simulink model "controller"  (Simulink 7.3)
settings: Solver=FixedStepDiscrete  StartTime=0.0  StopTime=inf  FixedStep=900  RelTol=1e-3
libraries: simulink x6
settings Model: Creator=mwetter  LastModifiedBy=mwetter  ExtModeAutoUpdateStatusClock=off
settings OptimizationCC: InitFltsAndDblsToZero=on
settings DebuggingCC: SaveWithParameterizedLinksMsg=none
settings GRTTargetCC: TargetFcnLib=ansi_tfl_tmw.mat

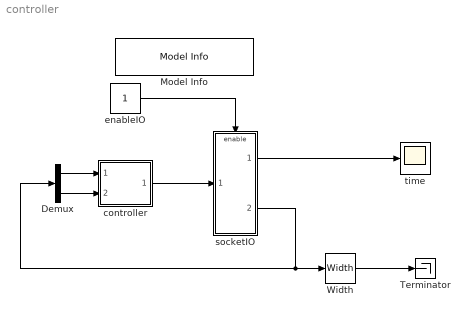
== system controller ==
  Demux : Demux  Outputs=2
  Model Info : simulink/Model-Wide Utilities/Model Info  SystemSampleTime=-1  InitialBlockCM=None  BlockCM=None  Frame=off  DisplayStringWithTags=|  HorizontalTextAlignment=Left  LeftAlignmentValue=0.02  SourceBlockDiagram=controller  TagMaxNumber=20
      | Model Info
      | % Set to 1 to enable IO
  Terminator : Terminator
  Width : Width  DataType=int16
  controller : Subsystem
  enableIO : Constant  OutDataType=sfix(16)  OutScaling=2^0
  socketIO : Subsystem
  time : Scope
  wires:
  socketIO/2(dblOut) -> Width/1, Demux/1
  socketIO/1(simTim) -> time/1
  Width/1 -> Terminator/1
  enableIO/1 -> socketIO/Enable
  Demux/1 -> controller/1(time)
  Demux/2 -> controller/2(TOut)
  controller/1(TSet) -> socketIO/1(dblIn)

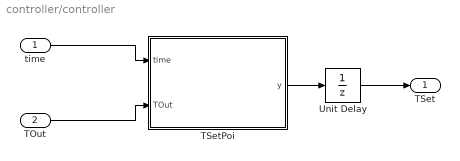
== system controller/controller ==
  time : Inport
  TOut : Inport  Port=2
  TSetPoi : Subsystem
  Unit Delay : UnitDelay  X0=[20, 25]  SampleTime=-1
  TSet : Outport
  wires:
  time/1 -> TSetPoi/1(time)
  TOut/1 -> TSetPoi/2(TOut)
  Unit Delay/1 -> TSet/1
  TSetPoi/1(y) -> Unit Delay/1

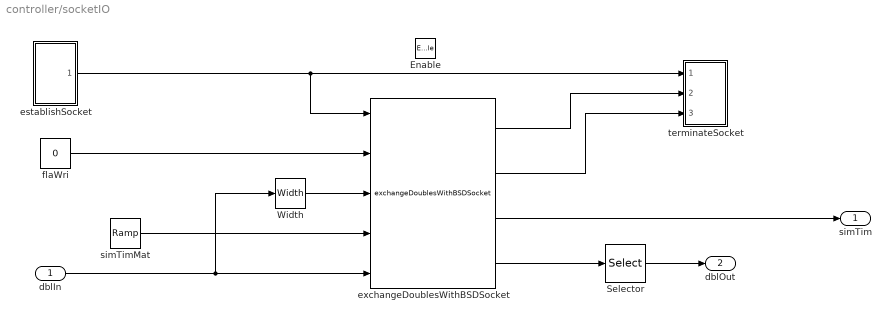
== system controller/socketIO ==
  dblIn : Inport
  Enable : EnablePort
  Selector : Selector  InputPortWidth=128  IndexOptions=Index vector (dialog)  Indices=[1 2]  OutputSizes=1
  Width : Width  DataType=int16
  establishSocket : Subsystem  TreatAsAtomicUnit=on
  exchangeDoublesWithBSDSocket : S-Function  FunctionName=exchangeDoublesWithBSDSocket  EnableBusSupport=off  mask(Legacy Function){SFunctionSpec=int16 y1 = exchangeDoublesWithBSDSocket(int16 u1[1], int16 u2[1], int16 y2[1], double u3[1], double u4[], double y3[1], double y4[50]), ShowSpec=off}
      mask prompts: ShowSpec "Display function specification"
      mask help:
      | This block allows the user to call the following C function(s) in Simulink:
      |
      |  InitializeConditionsFcn: none
      |
      |  StartFcn: none
      |
      |  OutputFcn: int16 y1 = exchangeDoublesWithBSDSocket(int16 u1[1], int16 u2[1], int16 y2[1], double u3[1], double u4[], double y3[1], double y4[50])
      |
      |  TerminateFcn: none
      mask CallbackString:
      | |if strcmp(get_param(gcbh, 'ShowSpec'), 'on')
      |   set_param(gcbh, 'MaskDisplay', sprintf('fprintf(''%s'');', get_param(gcbh, 'SFunctionSpec')));
      | else
      |   set_param(gcbh, 'MaskDisplay', sprintf('fprintf(''%s'');', get_param(gcbh, 'FunctionName')));
      | end
      mask Display: fprintf('exchangeDoublesWithBSDSocket');
  flaWri : Constant  Value=0  OutDataTypeMode=int16  OutDataType=sfix(16)  OutScaling=2^0  OutDataTypeStr=int16
  simTimMat : simulink/Sources/Ramp  SystemSampleTime=-1  slope=1  start=0  X0=0
  terminateSocket : Subsystem
  simTim : Outport
  dblOut : Outport  Port=2
  wires:
  establishSocket/1(socketFD) -> exchangeDoublesWithBSDSocket/1, terminateSocket/1(sockfd)
  flaWri/1 -> exchangeDoublesWithBSDSocket/2
  exchangeDoublesWithBSDSocket/3 -> simTim/1
  dblIn/1 -> exchangeDoublesWithBSDSocket/5, Width/1
  simTimMat/1 -> exchangeDoublesWithBSDSocket/4
  Width/1 -> exchangeDoublesWithBSDSocket/3
  Selector/1 -> dblOut/1
  exchangeDoublesWithBSDSocket/4 -> Selector/1
  exchangeDoublesWithBSDSocket/1 -> terminateSocket/2(excRetVal)
  exchangeDoublesWithBSDSocket/2 -> terminateSocket/3(excFlaRea)

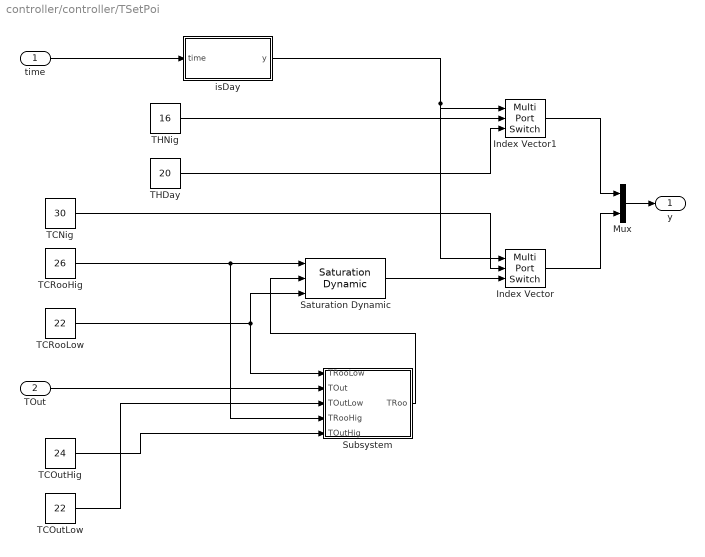
== system controller/controller/TSetPoi ==
  time : Inport  OutDataType=sfix(16)  OutScaling=2^0
  TOut : Inport  Port=2  OutDataType=sfix(16)  OutScaling=2^0
  Index Vector : MultiPortSwitch  Inputs=2  zeroidx=on  OutDataType=sfix(16)  OutScaling=2^0
  Index Vector1 : MultiPortSwitch  Inputs=2  zeroidx=on  OutDataType=sfix(16)  OutScaling=2^0
  Mux : Mux  Inputs=2
  Saturation Dynamic : simulink/Discontinuities/Saturation Dynamic  SystemSampleTime=-1  OutMin=[]  OutMax=[]  OutDataTypeStr=Inherit: Same as second input  OutDataType=sfix(16)  OutScaling=2^-10  DoSatur=off
  Subsystem : Subsystem
  TCNig : Constant  Value=30  OutDataType=sfix(16)  OutScaling=2^0
  TCOutHig : Constant  Value=24  OutDataType=sfix(16)  OutScaling=2^0
  TCOutLow : Constant  Value=22  OutDataType=sfix(16)  OutScaling=2^0
  TCRooHig : Constant  Value=26  OutDataType=sfix(16)  OutScaling=2^0
  TCRooLow : Constant  Value=22  OutDataType=sfix(16)  OutScaling=2^0
  THDay : Constant  Value=20  OutDataType=sfix(16)  OutScaling=2^0
  THNig : Constant  Value=16  OutDataType=sfix(16)  OutScaling=2^0
  isDay : Subsystem
  y : Outport  OutDataType=sfix(16)  OutScaling=2^0
  wires:
  TOut/1 -> Subsystem/2(TOut)
  TCOutLow/1 -> Subsystem/3(TOutLow)
  TCOutHig/1 -> Subsystem/5(TOutHig)
  TCRooHig/1 -> Saturation Dynamic/1, Subsystem/4(TRooHig)
  TCRooLow/1 -> Saturation Dynamic/3, Subsystem/1(TRooLow)
  time/1 -> isDay/1(time)
  isDay/1(y) -> Index Vector/1, Index Vector1/1
  TCNig/1 -> Index Vector/2
  Subsystem/1(TRoo) -> Saturation Dynamic/2
  Saturation Dynamic/1 -> Index Vector/3
  THNig/1 -> Index Vector1/2
  THDay/1 -> Index Vector1/3
  Index Vector1/1 -> Mux/1
  Index Vector/1 -> Mux/2
  Mux/1 -> y/1

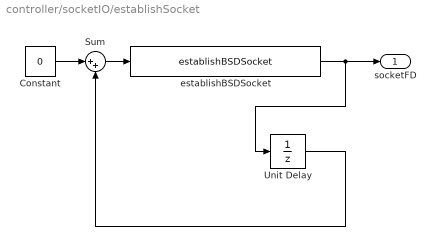
== system controller/socketIO/establishSocket ==
  Constant : Constant  Value=0  OutDataTypeMode=int16  OutDataType=sfix(16)  OutScaling=2^0  OutDataTypeStr=int16
  Sum : Sum  Inputs=|++  OutDataType=sfix(16)  OutScaling=2^0
  Unit Delay : UnitDelay  SampleTime=-1
  establishBSDSocket : S-Function  FunctionName=establishBSDSocket  EnableBusSupport=off  mask(Legacy Function){SFunctionSpec=int16 y1 = establishBSDSocket(void), ShowSpec=on}
      mask prompts: ShowSpec "Display function specification"
      mask help:
      | This block allows the user to call the following C function(s) in Simulink:
      |
      |  InitializeConditionsFcn: none
      |
      |  StartFcn: none
      |
      |  OutputFcn: int16 y1 = establishBSDSocket(void)
      |
      |  TerminateFcn: none
      mask CallbackString:
      | |if strcmp(get_param(gcbh, 'ShowSpec'), 'on')
      |   set_param(gcbh, 'MaskDisplay', sprintf('fprintf(''%s'');', get_param(gcbh, 'SFunctionSpec')));
      | else
      |   set_param(gcbh, 'MaskDisplay', sprintf('fprintf(''%s'');', get_param(gcbh, 'FunctionName')));
      | end
      mask Display: fprintf('int16 y1 = establishBSDSocket(void)');
  socketFD : Outport
  wires:
  establishBSDSocket/1 -> socketFD/1, Unit Delay/1
  Unit Delay/1 -> Sum/2
  Constant/1 -> Sum/1
  Sum/1 -> establishBSDSocket/1

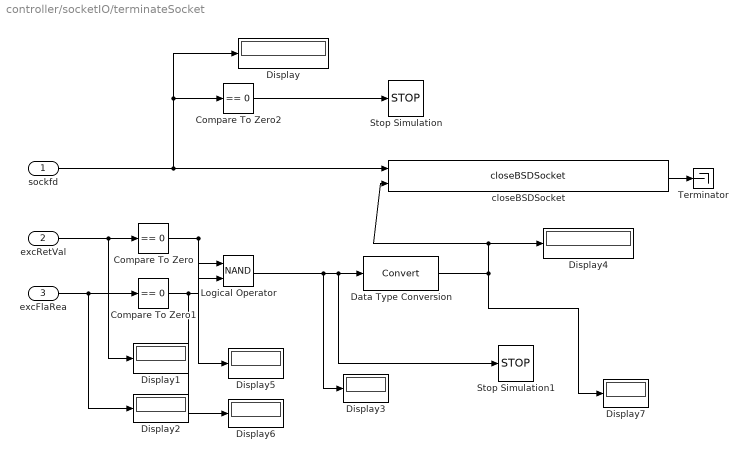
== system controller/socketIO/terminateSocket ==
  sockfd : Inport
  excRetVal : Inport  Port=2
  excFlaRea : Inport  Port=3
  Compare To Zero : simulink/Logic and Bit Operations/Compare To Zero  SystemSampleTime=-1  relop===  LogicOutDataTypeMode=uint8  ZeroCross=off
  Compare To Zero1 : simulink/Logic and Bit Operations/Compare To Zero  SystemSampleTime=-1  relop===  LogicOutDataTypeMode=uint8  ZeroCross=off
  Compare To Zero2 : simulink/Logic and Bit Operations/Compare To Zero  SystemSampleTime=-1  relop===  LogicOutDataTypeMode=boolean  ZeroCross=off
  Data Type Conversion : DataTypeConversion  OutDataType=sfix(16)  OutScaling=2^0
  Display{,1..7} (8 alike) : Display
  Logical Operator : Logic  Operator=NAND  AllPortsSameDT=off  OutDataTypeMode=boolean  OutDataTypeStr=boolean
  Stop Simulation : Stop
  Stop Simulation1 : Stop
  Terminator : Terminator
  closeBSDSocket : S-Function  FunctionName=closeBSDSocket  EnableBusSupport=off  mask(Legacy Function){SFunctionSpec=int16 y1 = closeBSDSocket(int16 u1[1], int16 u2[1]), ShowSpec=on}
      mask prompts: ShowSpec "Display function specification"
      mask help:
      | This block allows the user to call the following C function(s) in Simulink:
      |
      |  InitializeConditionsFcn: none
      |
      |  StartFcn: none
      |
      |  OutputFcn: int16 y1 = closeBSDSocket(int16 u1[1], int16 u2[1])
      |
      |  TerminateFcn: none
      mask CallbackString:
      | |if strcmp(get_param(gcbh, 'ShowSpec'), 'on')
      |   set_param(gcbh, 'MaskDisplay', sprintf('fprintf(''%s'');', get_param(gcbh, 'SFunctionSpec')));
      | else
      |   set_param(gcbh, 'MaskDisplay', sprintf('fprintf(''%s'');', get_param(gcbh, 'FunctionName')));
      | end
      mask Display: fprintf('int16 y1 = closeBSDSocket(int16 u1[1], int16 u2[1])');
  wires:
  sockfd/1 -> closeBSDSocket/1, Compare To Zero2/1, Display/1
  excRetVal/1 -> Compare To Zero/1, Display1/1
  excFlaRea/1 -> Compare To Zero1/1, Display2/1
  Compare To Zero/1 -> Logical Operator/1, Display5/1
  Compare To Zero1/1 -> Logical Operator/2, Display6/1
  Logical Operator/1 -> Display3/1, Data Type Conversion/1, Stop Simulation1/1
  Data Type Conversion/1 -> closeBSDSocket/2, Display4/1, Display7/1
  Compare To Zero2/1 -> Stop Simulation/1
  closeBSDSocket/1 -> Terminator/1

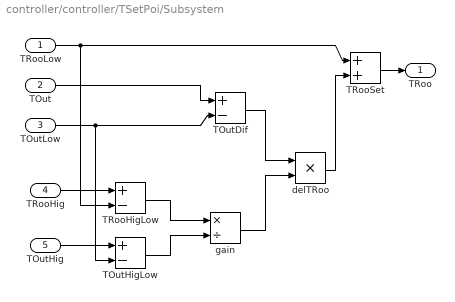
== system controller/controller/TSetPoi/Subsystem ==
  TRooLow : Inport
  TOut : Inport  Port=2
  TOutLow : Inport  Port=3
  TRooHig : Inport  Port=4
  TOutHig : Inport  Port=5
  TOutDif : Sum  Inputs=+-  OutDataType=sfix(16)  OutScaling=2^-10
  TOutHigLow : Sum  Inputs=+-  OutDataType=sfix(16)  OutScaling=2^-10
  TRooHigLow : Sum  Inputs=+-  OutDataType=sfix(16)  OutScaling=2^-10
  TRooSet : Sum  OutDataType=sfix(16)  OutScaling=2^-10
  delTRoo : Product  OutDataType=sfix(16)  OutScaling=2^0  RndMeth=Zero
  gain : Product  Inputs=*/  OutDataType=sfix(16)  OutScaling=2^-10
  TRoo : Outport
  wires:
  TRooHigLow/1 -> gain/1
  TOutHigLow/1 -> gain/2
  TOutDif/1 -> delTRoo/1
  gain/1 -> delTRoo/2
  delTRoo/1 -> TRooSet/2
  TRooLow/1 -> TRooSet/1, TRooHigLow/2
  TOutLow/1 -> TOutDif/2, TOutHigLow/2
  TRooHig/1 -> TRooHigLow/1
  TOutHig/1 -> TOutHigLow/1
  TRooSet/1 -> TRoo/1
  TOut/1 -> TOutDif/1

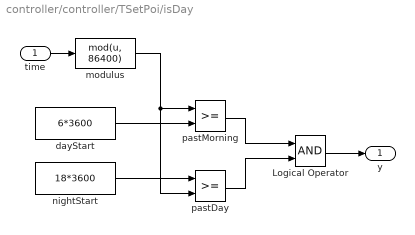
== system controller/controller/TSetPoi/isDay ==
  time : Inport
  Logical Operator : Logic  AllPortsSameDT=off  OutDataTypeMode=boolean  OutDataTypeStr=boolean
  dayStart : Constant  Value=6*3600  OutDataType=sfix(16)  OutScaling=2^0
  modulus : MATLABFcn  MATLABFcn=mod(u, 86400)
  nightStart : Constant  Value=18*3600  OutDataType=sfix(16)  OutScaling=2^0
  pastDay : RelationalOperator  LogicOutDataTypeMode=boolean  OutDataTypeStr=boolean
  pastMorning : RelationalOperator  LogicOutDataTypeMode=boolean  OutDataTypeStr=boolean
  y : Outport
  wires:
  time/1 -> modulus/1
  modulus/1 -> pastMorning/1, pastDay/2
  dayStart/1 -> pastMorning/2
  nightStart/1 -> pastDay/1
  pastMorning/1 -> Logical Operator/1
  pastDay/1 -> Logical Operator/2
  Logical Operator/1 -> y/1
